simulink model "TST_CoETS_TrqCalc"  (R2016b)
settings: Solver=FixedStepDiscrete  StartTime=0.0  StopTime=simTime  FixedStep=sampleTime  RelTol=1e-3
values from neighbouring files (symbols this model uses):
  testCase = 1    [initTST_CoETS_TrqCalc_001.m]    (also in initTST_CoETS_TrqCalc_002.m = 2; initTST_CoETS_TrqCalc_003.m = 3)
libraries: simulink x52, UnitTest_Lib x48
(part 1 of 2)
settings Model: Creator=zhengjinyan  LastModifiedBy=zhengjinyan
settings DebuggingCC: SignalRangeChecking=error

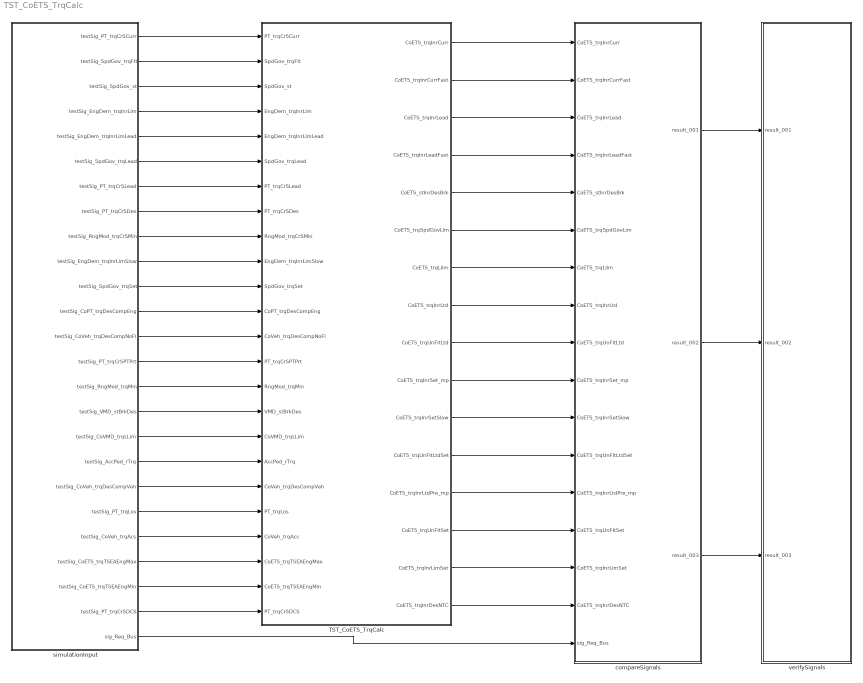
== system TST_CoETS_TrqCalc ==
  TST_CoETS_TrqCalc : Subsystem
  compareSignals : Subsystem
  simulationInput : Subsystem
  verifySignals : Subsystem
  wires:
  simulationInput/1(testSig_PT_trqCrSCurr) -> TST_CoETS_TrqCalc/1(PT_trqCrSCurr)
  simulationInput/2(testSig_SpdGov_trqFlt) -> TST_CoETS_TrqCalc/2(SpdGov_trqFlt)
  simulationInput/3(testSig_SpdGov_st) -> TST_CoETS_TrqCalc/3(SpdGov_st)
  simulationInput/4(testSig_EngDem_trqInrLim) -> TST_CoETS_TrqCalc/4(EngDem_trqInrLim)
  simulationInput/5(testSig_EngDem_trqInrLimLead) -> TST_CoETS_TrqCalc/5(EngDem_trqInrLimLead)
  simulationInput/6(testSig_SpdGov_trqLead) -> TST_CoETS_TrqCalc/6(SpdGov_trqLead)
  simulationInput/7(testSig_PT_trqCrSLead) -> TST_CoETS_TrqCalc/7(PT_trqCrSLead)
  simulationInput/8(testSig_PT_trqCrSDes) -> TST_CoETS_TrqCalc/8(PT_trqCrSDes)
  simulationInput/9(testSig_RngMod_trqCrSMin) -> TST_CoETS_TrqCalc/9(RngMod_trqCrSMin)
  simulationInput/10(testSig_EngDem_trqInrLimSlow) -> TST_CoETS_TrqCalc/10(EngDem_trqInrLimSlow)
  simulationInput/11(testSig_SpdGov_trqSet) -> TST_CoETS_TrqCalc/11(SpdGov_trqSet)
  simulationInput/12(testSig_CoPT_trqDesCompEng) -> TST_CoETS_TrqCalc/12(CoPT_trqDesCompEng)
  simulationInput/13(testSig_CoVeh_trqDesCompNoFl) -> TST_CoETS_TrqCalc/13(CoVeh_trqDesCompNoFl)
  simulationInput/14(testSig_PT_trqCrSPTPrt) -> TST_CoETS_TrqCalc/14(PT_trqCrSPTPrt)
  simulationInput/15(testSig_RngMod_trqMin) -> TST_CoETS_TrqCalc/15(RngMod_trqMin)
  simulationInput/16(testSig_VMD_stBrkDes) -> TST_CoETS_TrqCalc/16(VMD_stBrkDes)
  simulationInput/17(testSig_CoVMD_trqLLim) -> TST_CoETS_TrqCalc/17(CoVMD_trqLLim)
  simulationInput/18(testSig_AccPed_rTrq) -> TST_CoETS_TrqCalc/18(AccPed_rTrq)
  simulationInput/19(testSig_CoVeh_trqDesCompVeh) -> TST_CoETS_TrqCalc/19(CoVeh_trqDesCompVeh)
  simulationInput/20(testSig_PT_trqLos) -> TST_CoETS_TrqCalc/20(PT_trqLos)
  simulationInput/21(testSig_CoVeh_trqAcs) -> TST_CoETS_TrqCalc/21(CoVeh_trqAcs)
  simulationInput/22(testSig_CoETS_trqTSEAEngMax) -> TST_CoETS_TrqCalc/22(CoETS_trqTSEAEngMax)
  simulationInput/23(testSig_CoETS_trqTSEAEngMin) -> TST_CoETS_TrqCalc/23(CoETS_trqTSEAEngMin)
  simulationInput/24(testSig_PT_trqCrSDCS) -> TST_CoETS_TrqCalc/24(PT_trqCrSDCS)
  TST_CoETS_TrqCalc/1(CoETS_trqInrCurr) -> compareSignals/1(CoETS_trqInrCurr)
  TST_CoETS_TrqCalc/2(CoETS_trqInrCurrFast) -> compareSignals/2(CoETS_trqInrCurrFast)
  TST_CoETS_TrqCalc/3(CoETS_trqInrLead) -> compareSignals/3(CoETS_trqInrLead)
  TST_CoETS_TrqCalc/4(CoETS_trqInrLeadFast) -> compareSignals/4(CoETS_trqInrLeadFast)
  TST_CoETS_TrqCalc/5(CoETS_stInrDesBrk) -> compareSignals/5(CoETS_stInrDesBrk)
  TST_CoETS_TrqCalc/6(CoETS_trqSpdGovLim) -> compareSignals/6(CoETS_trqSpdGovLim)
  TST_CoETS_TrqCalc/7(CoETS_trqLlim) -> compareSignals/7(CoETS_trqLlim)
  TST_CoETS_TrqCalc/8(CoETS_trqInrLtd) -> compareSignals/8(CoETS_trqInrLtd)
  TST_CoETS_TrqCalc/9(CoETS_trqUnFltLtd) -> compareSignals/9(CoETS_trqUnFltLtd)
  TST_CoETS_TrqCalc/10(CoETS_trqInrSet_mp) -> compareSignals/10(CoETS_trqInrSet_mp)
  TST_CoETS_TrqCalc/11(CoETS_trqInrSetSlow) -> compareSignals/11(CoETS_trqInrSetSlow)
  TST_CoETS_TrqCalc/12(CoETS_trqUnFltLtdSet) -> compareSignals/12(CoETS_trqUnFltLtdSet)
  TST_CoETS_TrqCalc/13(CoETS_trqInrLtdPre_mp) -> compareSignals/13(CoETS_trqInrLtdPre_mp)
  TST_CoETS_TrqCalc/14(CoETS_trqUnFltSet) -> compareSignals/14(CoETS_trqUnFltSet)
  TST_CoETS_TrqCalc/15(CoETS_trqInrLimSet) -> compareSignals/15(CoETS_trqInrLimSet)
  TST_CoETS_TrqCalc/16(CoETS_trqInrDesNTC) -> compareSignals/16(CoETS_trqInrDesNTC)
  simulationInput/25(sig_Req_Bus) -> compareSignals/17(sig_Req_Bus)
  compareSignals/1(result_001) -> verifySignals/1(result_001)
  compareSignals/2(result_002) -> verifySignals/2(result_002)
  compareSignals/3(result_003) -> verifySignals/3(result_003)

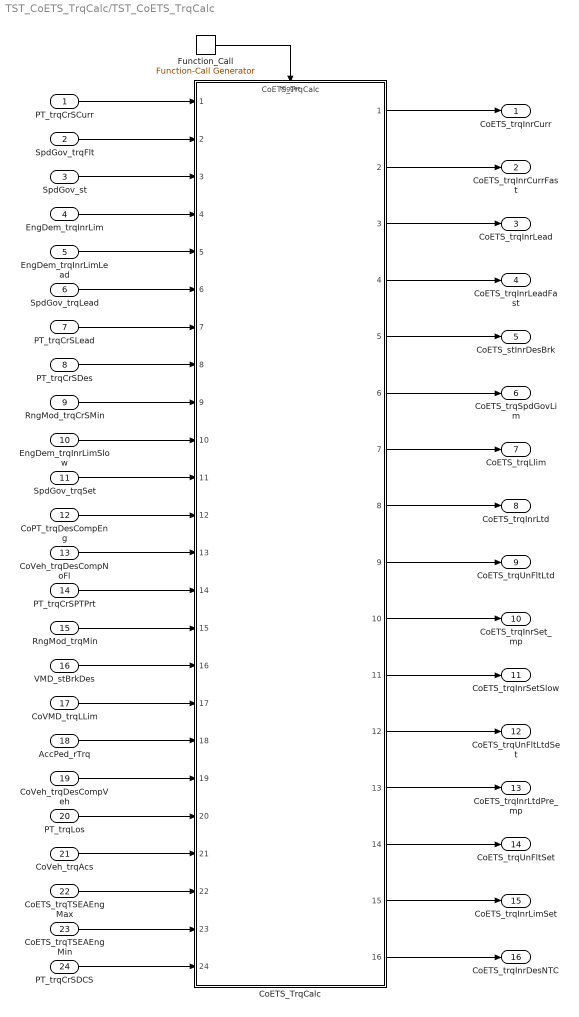
== system TST_CoETS_TrqCalc/TST_CoETS_TrqCalc ==
  PT_trqCrSCurr : Inport
  SpdGov_trqFlt : Inport  Port=2
  SpdGov_st : Inport  Port=3
  EngDem_trqInrLim : Inport  Port=4
  EngDem_trqInrLimLead : Inport  Port=5
  SpdGov_trqLead : Inport  Port=6
  PT_trqCrSLead : Inport  Port=7
  PT_trqCrSDes : Inport  Port=8
  RngMod_trqCrSMin : Inport  Port=9
  EngDem_trqInrLimSlow : Inport  Port=10
  SpdGov_trqSet : Inport  Port=11
  CoPT_trqDesCompEng : Inport  Port=12
  CoVeh_trqDesCompNoFl : Inport  Port=13
  PT_trqCrSPTPrt : Inport  Port=14
  RngMod_trqMin : Inport  Port=15
  VMD_stBrkDes : Inport  Port=16
  CoVMD_trqLLim : Inport  Port=17
  AccPed_rTrq : Inport  Port=18
  CoVeh_trqDesCompVeh : Inport  Port=19
  PT_trqLos : Inport  Port=20
  CoVeh_trqAcs : Inport  Port=21
  CoETS_trqTSEAEngMax : Inport  Port=22
  CoETS_trqTSEAEngMin : Inport  Port=23
  PT_trqCrSDCS : Inport  Port=24
  CoETS_TrqCalc : ModelReference  ModelNameDialog=CoETS_TrqCalc  SimulationMode=Normal  ModelReferenceVersion=1.10  TriggerPortName=function  TriggerPortTriggerType=function-call  TriggerPortStatesWhenEnabling=held
  Function_Call : simulink/Ports & Subsystems/Function-Call Generator  sample_time=sampleTime  numberOfIterations=1
  CoETS_trqInrCurr : Outport
  CoETS_trqInrCurrFast : Outport  Port=2
  CoETS_trqInrLead : Outport  Port=3
  CoETS_trqInrLeadFast : Outport  Port=4
  CoETS_stInrDesBrk : Outport  Port=5
  CoETS_trqSpdGovLim : Outport  Port=6
  CoETS_trqLlim : Outport  Port=7
  CoETS_trqInrLtd : Outport  Port=8
  CoETS_trqUnFltLtd : Outport  Port=9
  CoETS_trqInrSet_mp : Outport  Port=10
  CoETS_trqInrSetSlow : Outport  Port=11
  CoETS_trqUnFltLtdSet : Outport  Port=12
  CoETS_trqInrLtdPre_mp : Outport  Port=13
  CoETS_trqUnFltSet : Outport  Port=14
  CoETS_trqInrLimSet : Outport  Port=15
  CoETS_trqInrDesNTC : Outport  Port=16
  wires:
  Function_Call/1 -> CoETS_TrqCalc/Trigger
  PT_trqCrSCurr/1 -> CoETS_TrqCalc/1
  SpdGov_trqFlt/1 -> CoETS_TrqCalc/2
  SpdGov_st/1 -> CoETS_TrqCalc/3
  EngDem_trqInrLim/1 -> CoETS_TrqCalc/4
  EngDem_trqInrLimLead/1 -> CoETS_TrqCalc/5
  SpdGov_trqLead/1 -> CoETS_TrqCalc/6
  PT_trqCrSLead/1 -> CoETS_TrqCalc/7
  PT_trqCrSDes/1 -> CoETS_TrqCalc/8
  RngMod_trqCrSMin/1 -> CoETS_TrqCalc/9
  EngDem_trqInrLimSlow/1 -> CoETS_TrqCalc/10
  SpdGov_trqSet/1 -> CoETS_TrqCalc/11
  CoPT_trqDesCompEng/1 -> CoETS_TrqCalc/12
  CoVeh_trqDesCompNoFl/1 -> CoETS_TrqCalc/13
  PT_trqCrSPTPrt/1 -> CoETS_TrqCalc/14
  RngMod_trqMin/1 -> CoETS_TrqCalc/15
  VMD_stBrkDes/1 -> CoETS_TrqCalc/16
  CoVMD_trqLLim/1 -> CoETS_TrqCalc/17
  AccPed_rTrq/1 -> CoETS_TrqCalc/18
  CoVeh_trqDesCompVeh/1 -> CoETS_TrqCalc/19
  PT_trqLos/1 -> CoETS_TrqCalc/20
  CoVeh_trqAcs/1 -> CoETS_TrqCalc/21
  CoETS_trqTSEAEngMax/1 -> CoETS_TrqCalc/22
  CoETS_trqTSEAEngMin/1 -> CoETS_TrqCalc/23
  PT_trqCrSDCS/1 -> CoETS_TrqCalc/24
  CoETS_TrqCalc/1 -> CoETS_trqInrCurr/1
  CoETS_TrqCalc/2 -> CoETS_trqInrCurrFast/1
  CoETS_TrqCalc/3 -> CoETS_trqInrLead/1
  CoETS_TrqCalc/5 -> CoETS_stInrDesBrk/1
  CoETS_TrqCalc/6 -> CoETS_trqSpdGovLim/1
  CoETS_TrqCalc/7 -> CoETS_trqLlim/1
  CoETS_TrqCalc/8 -> CoETS_trqInrLtd/1
  CoETS_TrqCalc/9 -> CoETS_trqUnFltLtd/1
  CoETS_TrqCalc/10 -> CoETS_trqInrSet_mp/1
  CoETS_TrqCalc/11 -> CoETS_trqInrSetSlow/1
  CoETS_TrqCalc/12 -> CoETS_trqUnFltLtdSet/1
  CoETS_TrqCalc/13 -> CoETS_trqInrLtdPre_mp/1
  CoETS_TrqCalc/15 -> CoETS_trqInrLimSet/1
  CoETS_TrqCalc/16 -> CoETS_trqInrDesNTC/1
  CoETS_TrqCalc/4 -> CoETS_trqInrLeadFast/1
  CoETS_TrqCalc/14 -> CoETS_trqUnFltSet/1

== system TST_CoETS_TrqCalc/compareSignals ==
  CoETS_trqInrCurr : Inport
  CoETS_trqInrCurrFast : Inport  Port=2
  CoETS_trqInrLead : Inport  Port=3
  CoETS_trqInrLeadFast : Inport  Port=4
  CoETS_stInrDesBrk : Inport  Port=5
  CoETS_trqSpdGovLim : Inport  Port=6
  CoETS_trqLlim : Inport  Port=7
  CoETS_trqInrLtd : Inport  Port=8
  CoETS_trqUnFltLtd : Inport  Port=9
  CoETS_trqInrSet_mp : Inport  Port=10
  CoETS_trqInrSetSlow : Inport  Port=11
  CoETS_trqUnFltLtdSet : Inport  Port=12
  CoETS_trqInrLtdPre_mp : Inport  Port=13
  CoETS_trqUnFltSet : Inport  Port=14
  CoETS_trqInrLimSet : Inport  Port=15
  CoETS_trqInrDesNTC : Inport  Port=16
  sig_Req_Bus : Inport  Port=17
  BC : BusCreator  Inputs=16
  CTC_001 : simulink/Logic and Bit Operations/Compare To Constant  relop===  const=1  OutDataTypeStr=boolean
  CTC_002 : simulink/Logic and Bit Operations/Compare To Constant  relop===  const=2  OutDataTypeStr=boolean
  CTC_003 : simulink/Logic and Bit Operations/Compare To Constant  relop===  const=3  OutDataTypeStr=boolean
  Requirement_001 : Subsystem
  Requirement_002 : Subsystem
  Requirement_003 : Subsystem
  TC_001 : Constant  Value=testCase
  TC_002 : Constant  Value=testCase
  TC_003 : Constant  Value=testCase
  result_001 : Outport
  result_002 : Outport  Port=2
  result_003 : Outport  Port=3
  wires:
  CoETS_trqInrCurr/1 -> BC/1  "CoETS_trqInrCurr"
  CoETS_trqInrCurrFast/1 -> BC/2  "CoETS_trqInrCurrFast"
  CoETS_trqInrLead/1 -> BC/3  "CoETS_trqInrLead"
  CoETS_trqInrLeadFast/1 -> BC/4  "CoETS_trqInrLeadFast"
  CoETS_stInrDesBrk/1 -> BC/5  "CoETS_stInrDesBrk"
  CoETS_trqSpdGovLim/1 -> BC/6  "CoETS_trqSpdGovLim"
  CoETS_trqLlim/1 -> BC/7  "CoETS_trqLlim"
  CoETS_trqInrLtd/1 -> BC/8  "CoETS_trqInrLtd"
  CoETS_trqUnFltLtd/1 -> BC/9  "CoETS_trqUnFltLtd"
  CoETS_trqInrSet_mp/1 -> BC/10  "CoETS_trqInrSet_mp"
  CoETS_trqInrSetSlow/1 -> BC/11  "CoETS_trqInrSetSlow"
  CoETS_trqUnFltLtdSet/1 -> BC/12  "CoETS_trqUnFltLtdSet"
  CoETS_trqInrLtdPre_mp/1 -> BC/13  "CoETS_trqInrLtdPre_mp"
  CoETS_trqUnFltSet/1 -> BC/14  "CoETS_trqUnFltSet"
  CoETS_trqInrLimSet/1 -> BC/15  "CoETS_trqInrLimSet"
  CoETS_trqInrDesNTC/1 -> BC/16  "CoETS_trqInrDesNTC"
  TC_001/1 -> CTC_001/1
  CTC_001/1 -> Requirement_001/Enable
  sig_Req_Bus/1 -> Requirement_001/2(sig_Req_Bus), Requirement_002/2(sig_Req_Bus), Requirement_003/2(sig_Req_Bus)
  BC/1 -> Requirement_002/1(sig_Result_Bus), Requirement_003/1(sig_Result_Bus), Requirement_001/1(sig_Result_Bus)
  Requirement_001/1(result) -> result_001/1
  TC_002/1 -> CTC_002/1
  CTC_002/1 -> Requirement_002/Enable
  Requirement_002/1(result) -> result_002/1
  TC_003/1 -> CTC_003/1
  CTC_003/1 -> Requirement_003/Enable
  Requirement_003/1(result) -> result_003/1

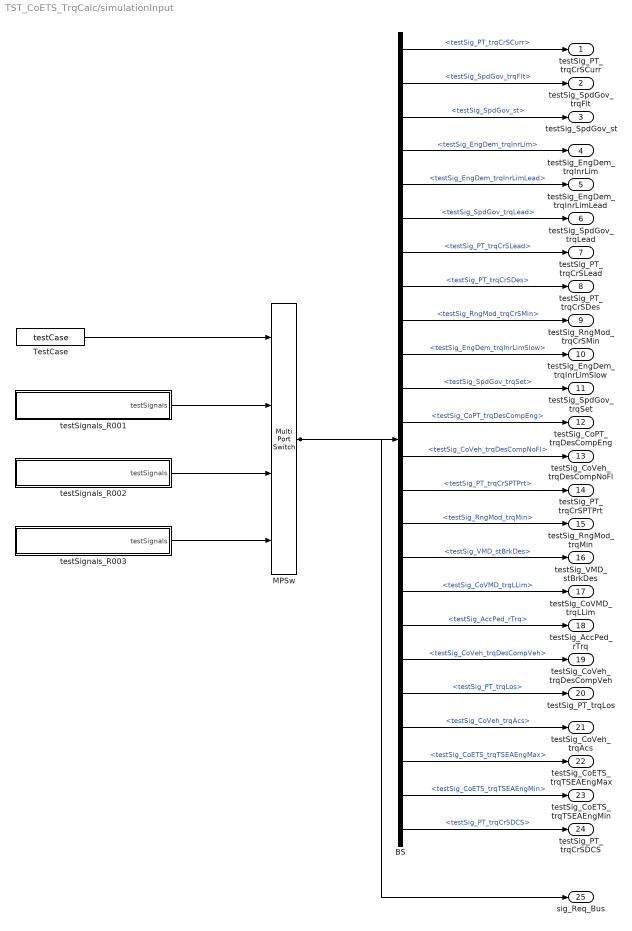
== system TST_CoETS_TrqCalc/simulationInput ==
  BS : BusSelector  OutputSignals=testSig_PT_trqCrSCurr,testSig_SpdGov_trqFlt,testSig_SpdGov_st,testSig_EngDem_trqInrLim,testSig_EngDem_trqInrLimLead,testSig_SpdGov_trqLead,testSig_PT_trqCrSLead,testSig_PT_trqCrSDes,testSig_RngMod_trqCrSMin,testSig_EngDem_trqInrLimSlow,testSig_SpdGov_trqSet,testSig_CoPT_trqDesCompEng,testSig_CoVeh_trqDesCompNoFl,testSig_PT_trqCrSPTPrt,testSig_RngMod_trqMin,testSig_VMD_stBrkDes,testSig_CoVMD_trqLLim,testSig_AccPed_rTrq,testSig_CoVeh_trqDesCompVeh,testSig_PT_trqLos,testSig_CoVeh_trqAcs,testSig_CoETS_trqTSEAEngMax,testSig_CoETS_trqTSEAEngMin,testSig_PT_trqCrSDCS
  MPSw : MultiPortSwitch  SaturateOnIntegerOverflow=on  InputSameDT=on
  TestCase : Constant  Value=testCase
  testSignals_R001 : Subsystem
  testSignals_R002 : Subsystem
  testSignals_R003 : Subsystem
  testSig_PT_trqCrSCurr : Outport
  testSig_SpdGov_trqFlt : Outport  Port=2
  testSig_SpdGov_st : Outport  Port=3
  testSig_EngDem_trqInrLim : Outport  Port=4
  testSig_EngDem_trqInrLimLead : Outport  Port=5
  testSig_SpdGov_trqLead : Outport  Port=6
  testSig_PT_trqCrSLead : Outport  Port=7
  testSig_PT_trqCrSDes : Outport  Port=8
  testSig_RngMod_trqCrSMin : Outport  Port=9
  testSig_EngDem_trqInrLimSlow : Outport  Port=10
  testSig_SpdGov_trqSet : Outport  Port=11
  testSig_CoPT_trqDesCompEng : Outport  Port=12
  testSig_CoVeh_trqDesCompNoFl : Outport  Port=13
  testSig_PT_trqCrSPTPrt : Outport  Port=14
  testSig_RngMod_trqMin : Outport  Port=15
  testSig_VMD_stBrkDes : Outport  Port=16
  testSig_CoVMD_trqLLim : Outport  Port=17
  testSig_AccPed_rTrq : Outport  Port=18
  testSig_CoVeh_trqDesCompVeh : Outport  Port=19
  testSig_PT_trqLos : Outport  Port=20
  testSig_CoVeh_trqAcs : Outport  Port=21
  testSig_CoETS_trqTSEAEngMax : Outport  Port=22
  testSig_CoETS_trqTSEAEngMin : Outport  Port=23
  testSig_PT_trqCrSDCS : Outport  Port=24
  sig_Req_Bus : Outport  Port=25
  wires:
  BS/1 -> testSig_PT_trqCrSCurr/1  "<testSig_PT_trqCrSCurr>"
  BS/2 -> testSig_SpdGov_trqFlt/1  "<testSig_SpdGov_trqFlt>"
  BS/3 -> testSig_SpdGov_st/1  "<testSig_SpdGov_st>"
  BS/4 -> testSig_EngDem_trqInrLim/1  "<testSig_EngDem_trqInrLim>"
  BS/5 -> testSig_EngDem_trqInrLimLead/1  "<testSig_EngDem_trqInrLimLead>"
  BS/6 -> testSig_SpdGov_trqLead/1  "<testSig_SpdGov_trqLead>"
  BS/7 -> testSig_PT_trqCrSLead/1  "<testSig_PT_trqCrSLead>"
  BS/8 -> testSig_PT_trqCrSDes/1  "<testSig_PT_trqCrSDes>"
  BS/9 -> testSig_RngMod_trqCrSMin/1  "<testSig_RngMod_trqCrSMin>"
  BS/10 -> testSig_EngDem_trqInrLimSlow/1  "<testSig_EngDem_trqInrLimSlow>"
  BS/11 -> testSig_SpdGov_trqSet/1  "<testSig_SpdGov_trqSet>"
  BS/12 -> testSig_CoPT_trqDesCompEng/1  "<testSig_CoPT_trqDesCompEng>"
  BS/13 -> testSig_CoVeh_trqDesCompNoFl/1  "<testSig_CoVeh_trqDesCompNoFl>"
  BS/14 -> testSig_PT_trqCrSPTPrt/1  "<testSig_PT_trqCrSPTPrt>"
  BS/15 -> testSig_RngMod_trqMin/1  "<testSig_RngMod_trqMin>"
  BS/16 -> testSig_VMD_stBrkDes/1  "<testSig_VMD_stBrkDes>"
  BS/17 -> testSig_CoVMD_trqLLim/1  "<testSig_CoVMD_trqLLim>"
  BS/18 -> testSig_AccPed_rTrq/1  "<testSig_AccPed_rTrq>"
  BS/19 -> testSig_CoVeh_trqDesCompVeh/1  "<testSig_CoVeh_trqDesCompVeh>"
  BS/20 -> testSig_PT_trqLos/1  "<testSig_PT_trqLos>"
  BS/21 -> testSig_CoVeh_trqAcs/1  "<testSig_CoVeh_trqAcs>"
  BS/22 -> testSig_CoETS_trqTSEAEngMax/1  "<testSig_CoETS_trqTSEAEngMax>"
  BS/23 -> testSig_CoETS_trqTSEAEngMin/1  "<testSig_CoETS_trqTSEAEngMin>"
  BS/24 -> testSig_PT_trqCrSDCS/1  "<testSig_PT_trqCrSDCS>"
  MPSw/1 -> BS/1, sig_Req_Bus/1
  TestCase/1 -> MPSw/1
  testSignals_R001/1(testSignals) -> MPSw/2
  testSignals_R002/1(testSignals) -> MPSw/3
  testSignals_R003/1(testSignals) -> MPSw/4

== system TST_CoETS_TrqCalc/verifySignals ==
  result_001 : Inport
  result_002 : Inport  Port=2
  result_003 : Inport  Port=3
  Assertion_001 : Assertion  Enabled=off
  Assertion_002 : Assertion  Enabled=off
  Assertion_003 : Assertion  Enabled=off
  wires:
  result_001/1 -> Assertion_001/1
  result_002/1 -> Assertion_002/1
  result_003/1 -> Assertion_003/1

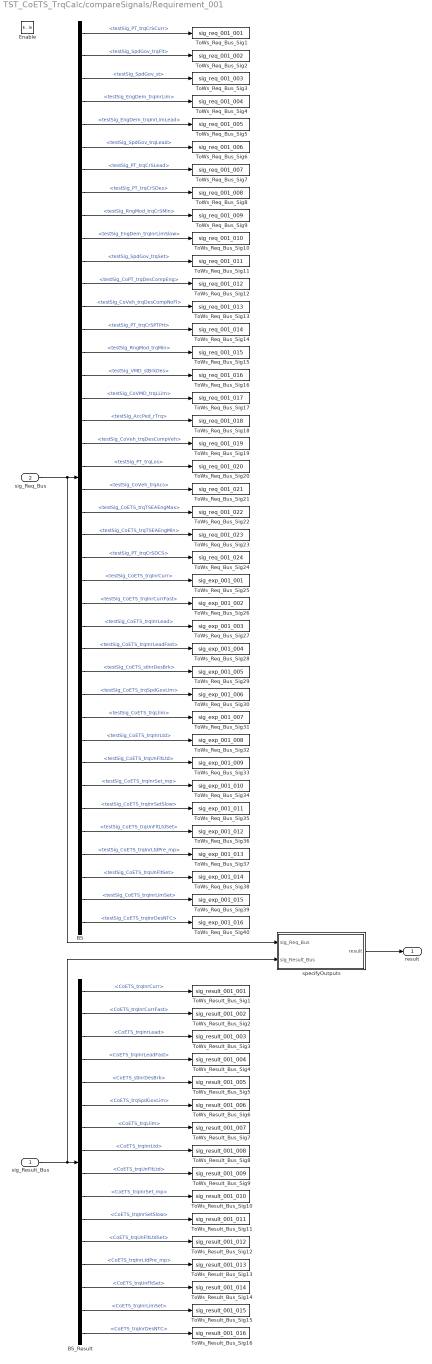
== system TST_CoETS_TrqCalc/compareSignals/Requirement_001 ==
  sig_Result_Bus : Inport
  sig_Req_Bus : Inport  Port=2
  Enable : EnablePort
  BS : BusSelector  OutputSignals=testSig_PT_trqCrSCurr,testSig_SpdGov_trqFlt,testSig_SpdGov_st,testSig_EngDem_trqInrLim,testSig_EngDem_trqInrLimLead,testSig_SpdGov_trqLead,testSig_PT_trqCrSLead,testSig_PT_trqCrSDes,testSig_RngMod_trqCrSMin,testSig_EngDem_trqInrLimSlow,testSig_SpdGov_trqSet,testSig_CoPT_trqDesCompEng,testSig_CoVeh_trqDesCompNoFl,testSig_PT_trqCrSPTPrt,testSig_RngMod_trqMin,testSig_VMD_stBrkDes,testSig_CoVMD_trqLLim,testSig_AccPed_rTrq,testSig_CoVeh_trqDesCompVeh,testSig_PT_trqLos,testSig_CoVeh_trqAcs,testSig_CoETS_trqTSEAEngMax,testSig_CoETS_trqTSEAEngMin,testSig_PT_trqCrSDCS,testSig_CoETS_trqInrCurr,testSig_CoETS_trqInrCurrFast,testSig_CoETS_trqInrLead,testSig_CoETS_trqInrLeadFast,testSig_CoETS_stInrDesBrk,testSig_CoETS_trqSpdGovLim,testSig_CoETS_trqLlim,testSig_CoETS_trqInrLtd,testSig_CoETS_trqUnFltLtd,testSig_CoETS_trqInrSet_mp,testSig_CoETS_trqInrSetSlow,testSig_CoETS_trqUnFltLtdSet,testSig_CoETS_trqInrLtdPre_mp,testSig_CoETS_trqUnFltSet,testSig_CoETS_trqInrLimSet,testSig_CoETS_trqInrDesNTC
  BS_Result : BusSelector  OutputSignals=CoETS_trqInrCurr,CoETS_trqInrCurrFast,CoETS_trqInrLead,CoETS_trqInrLeadFast,CoETS_stInrDesBrk,CoETS_trqSpdGovLim,CoETS_trqLlim,CoETS_trqInrLtd,CoETS_trqUnFltLtd,CoETS_trqInrSet_mp,CoETS_trqInrSetSlow,CoETS_trqUnFltLtdSet,CoETS_trqInrLtdPre_mp,CoETS_trqUnFltSet,CoETS_trqInrLimSet,CoETS_trqInrDesNTC
  ToWs_Req_Bus_Sig1 : ToWorkspace  VariableName=sig_req_001_001  SaveFormat=Structure With Time
  ToWs_Req_Bus_Sig10 : ToWorkspace  VariableName=sig_req_001_010  SaveFormat=Structure With Time
  ToWs_Req_Bus_Sig11 : ToWorkspace  VariableName=sig_req_001_011  SaveFormat=Structure With Time
  ToWs_Req_Bus_Sig12 : ToWorkspace  VariableName=sig_req_001_012  SaveFormat=Structure With Time
  ToWs_Req_Bus_Sig13 : ToWorkspace  VariableName=sig_req_001_013  SaveFormat=Structure With Time
  ToWs_Req_Bus_Sig14 : ToWorkspace  VariableName=sig_req_001_014  SaveFormat=Structure With Time
  ToWs_Req_Bus_Sig15 : ToWorkspace  VariableName=sig_req_001_015  SaveFormat=Structure With Time
  ToWs_Req_Bus_Sig16 : ToWorkspace  VariableName=sig_req_001_016  SaveFormat=Structure With Time
  ToWs_Req_Bus_Sig17 : ToWorkspace  VariableName=sig_req_001_017  SaveFormat=Structure With Time
  ToWs_Req_Bus_Sig18 : ToWorkspace  VariableName=sig_req_001_018  SaveFormat=Structure With Time
  ToWs_Req_Bus_Sig19 : ToWorkspace  VariableName=sig_req_001_019  SaveFormat=Structure With Time
  ToWs_Req_Bus_Sig2 : ToWorkspace  VariableName=sig_req_001_002  SaveFormat=Structure With Time
  ToWs_Req_Bus_Sig20 : ToWorkspace  VariableName=sig_req_001_020  SaveFormat=Structure With Time
  ToWs_Req_Bus_Sig21 : ToWorkspace  VariableName=sig_req_001_021  SaveFormat=Structure With Time
  ToWs_Req_Bus_Sig22 : ToWorkspace  VariableName=sig_req_001_022  SaveFormat=Structure With Time
  ToWs_Req_Bus_Sig23 : ToWorkspace  VariableName=sig_req_001_023  SaveFormat=Structure With Time
  ToWs_Req_Bus_Sig24 : ToWorkspace  VariableName=sig_req_001_024  SaveFormat=Structure With Time
  ToWs_Req_Bus_Sig25 : ToWorkspace  VariableName=sig_exp_001_001  SaveFormat=Structure With Time
  ToWs_Req_Bus_Sig26 : ToWorkspace  VariableName=sig_exp_001_002  SaveFormat=Structure With Time
  ToWs_Req_Bus_Sig27 : ToWorkspace  VariableName=sig_exp_001_003  SaveFormat=Structure With Time
  ToWs_Req_Bus_Sig28 : ToWorkspace  VariableName=sig_exp_001_004  SaveFormat=Structure With Time
  ToWs_Req_Bus_Sig29 : ToWorkspace  VariableName=sig_exp_001_005  SaveFormat=Structure With Time
  ToWs_Req_Bus_Sig3 : ToWorkspace  VariableName=sig_req_001_003  SaveFormat=Structure With Time
  ToWs_Req_Bus_Sig30 : ToWorkspace  VariableName=sig_exp_001_006  SaveFormat=Structure With Time
  ToWs_Req_Bus_Sig31 : ToWorkspace  VariableName=sig_exp_001_007  SaveFormat=Structure With Time
  ToWs_Req_Bus_Sig32 : ToWorkspace  VariableName=sig_exp_001_008  SaveFormat=Structure With Time
  ToWs_Req_Bus_Sig33 : ToWorkspace  VariableName=sig_exp_001_009  SaveFormat=Structure With Time
  ToWs_Req_Bus_Sig34 : ToWorkspace  VariableName=sig_exp_001_010  SaveFormat=Structure With Time
  ToWs_Req_Bus_Sig35 : ToWorkspace  VariableName=sig_exp_001_011  SaveFormat=Structure With Time
  ToWs_Req_Bus_Sig36 : ToWorkspace  VariableName=sig_exp_001_012  SaveFormat=Structure With Time
  ToWs_Req_Bus_Sig37 : ToWorkspace  VariableName=sig_exp_001_013  SaveFormat=Structure With Time
  ToWs_Req_Bus_Sig38 : ToWorkspace  VariableName=sig_exp_001_014  SaveFormat=Structure With Time
  ToWs_Req_Bus_Sig39 : ToWorkspace  VariableName=sig_exp_001_015  SaveFormat=Structure With Time
  ToWs_Req_Bus_Sig4 : ToWorkspace  VariableName=sig_req_001_004  SaveFormat=Structure With Time
  ToWs_Req_Bus_Sig40 : ToWorkspace  VariableName=sig_exp_001_016  SaveFormat=Structure With Time
  ToWs_Req_Bus_Sig5 : ToWorkspace  VariableName=sig_req_001_005  SaveFormat=Structure With Time
  ToWs_Req_Bus_Sig6 : ToWorkspace  VariableName=sig_req_001_006  SaveFormat=Structure With Time
  ToWs_Req_Bus_Sig7 : ToWorkspace  VariableName=sig_req_001_007  SaveFormat=Structure With Time
  ToWs_Req_Bus_Sig8 : ToWorkspace  VariableName=sig_req_001_008  SaveFormat=Structure With Time
  ToWs_Req_Bus_Sig9 : ToWorkspace  VariableName=sig_req_001_009  SaveFormat=Structure With Time
  ToWs_Result_Bus_Sig1 : ToWorkspace  VariableName=sig_result_001_001  SaveFormat=Structure With Time
  ToWs_Result_Bus_Sig10 : ToWorkspace  VariableName=sig_result_001_010  SaveFormat=Structure With Time
  ToWs_Result_Bus_Sig11 : ToWorkspace  VariableName=sig_result_001_011  SaveFormat=Structure With Time
  ToWs_Result_Bus_Sig12 : ToWorkspace  VariableName=sig_result_001_012  SaveFormat=Structure With Time
  ToWs_Result_Bus_Sig13 : ToWorkspace  VariableName=sig_result_001_013  SaveFormat=Structure With Time
  ToWs_Result_Bus_Sig14 : ToWorkspace  VariableName=sig_result_001_014  SaveFormat=Structure With Time
  ToWs_Result_Bus_Sig15 : ToWorkspace  VariableName=sig_result_001_015  SaveFormat=Structure With Time
  ToWs_Result_Bus_Sig16 : ToWorkspace  VariableName=sig_result_001_016  SaveFormat=Structure With Time
  ToWs_Result_Bus_Sig2 : ToWorkspace  VariableName=sig_result_001_002  SaveFormat=Structure With Time
  ToWs_Result_Bus_Sig3 : ToWorkspace  VariableName=sig_result_001_003  SaveFormat=Structure With Time
  ToWs_Result_Bus_Sig4 : ToWorkspace  VariableName=sig_result_001_004  SaveFormat=Structure With Time
  ToWs_Result_Bus_Sig5 : ToWorkspace  VariableName=sig_result_001_005  SaveFormat=Structure With Time
  ToWs_Result_Bus_Sig6 : ToWorkspace  VariableName=sig_result_001_006  SaveFormat=Structure With Time
  ToWs_Result_Bus_Sig7 : ToWorkspace  VariableName=sig_result_001_007  SaveFormat=Structure With Time
  ToWs_Result_Bus_Sig8 : ToWorkspace  VariableName=sig_result_001_008  SaveFormat=Structure With Time
  ToWs_Result_Bus_Sig9 : ToWorkspace  VariableName=sig_result_001_009  SaveFormat=Structure With Time
  specifyOutputs : Subsystem
  result : Outport
  wires:
  sig_Req_Bus/1 -> BS/1, specifyOutputs/1(sig_Req_Bus)
  BS/1 -> ToWs_Req_Bus_Sig1/1  "<testSig_PT_trqCrSCurr>"
  BS/2 -> ToWs_Req_Bus_Sig2/1  "<testSig_SpdGov_trqFlt>"
  BS/3 -> ToWs_Req_Bus_Sig3/1  "<testSig_SpdGov_st>"
  BS/4 -> ToWs_Req_Bus_Sig4/1  "<testSig_EngDem_trqInrLim>"
  BS/5 -> ToWs_Req_Bus_Sig5/1  "<testSig_EngDem_trqInrLimLead>"
  BS/6 -> ToWs_Req_Bus_Sig6/1  "<testSig_SpdGov_trqLead>"
  BS/7 -> ToWs_Req_Bus_Sig7/1  "<testSig_PT_trqCrSLead>"
  BS/8 -> ToWs_Req_Bus_Sig8/1  "<testSig_PT_trqCrSDes>"
  BS/9 -> ToWs_Req_Bus_Sig9/1  "<testSig_RngMod_trqCrSMin>"
  BS/10 -> ToWs_Req_Bus_Sig10/1  "<testSig_EngDem_trqInrLimSlow>"
  BS/11 -> ToWs_Req_Bus_Sig11/1  "<testSig_SpdGov_trqSet>"
  BS/12 -> ToWs_Req_Bus_Sig12/1  "<testSig_CoPT_trqDesCompEng>"
  BS/13 -> ToWs_Req_Bus_Sig13/1  "<testSig_CoVeh_trqDesCompNoFl>"
  BS/14 -> ToWs_Req_Bus_Sig14/1  "<testSig_PT_trqCrSPTPrt>"
  BS/15 -> ToWs_Req_Bus_Sig15/1  "<testSig_RngMod_trqMin>"
  BS/16 -> ToWs_Req_Bus_Sig16/1  "<testSig_VMD_stBrkDes>"
  BS/17 -> ToWs_Req_Bus_Sig17/1  "<testSig_CoVMD_trqLLim>"
  BS/18 -> ToWs_Req_Bus_Sig18/1  "<testSig_AccPed_rTrq>"
  BS/19 -> ToWs_Req_Bus_Sig19/1  "<testSig_CoVeh_trqDesCompVeh>"
  BS/20 -> ToWs_Req_Bus_Sig20/1  "<testSig_PT_trqLos>"
  BS/21 -> ToWs_Req_Bus_Sig21/1  "<testSig_CoVeh_trqAcs>"
  BS/22 -> ToWs_Req_Bus_Sig22/1  "<testSig_CoETS_trqTSEAEngMax>"
  BS/23 -> ToWs_Req_Bus_Sig23/1  "<testSig_CoETS_trqTSEAEngMin>"
  BS/24 -> ToWs_Req_Bus_Sig24/1  "<testSig_PT_trqCrSDCS>"
  BS/25 -> ToWs_Req_Bus_Sig25/1  "<testSig_CoETS_trqInrCurr>"
  BS/26 -> ToWs_Req_Bus_Sig26/1  "<testSig_CoETS_trqInrCurrFast>"
  BS/27 -> ToWs_Req_Bus_Sig27/1  "<testSig_CoETS_trqInrLead>"
  BS/28 -> ToWs_Req_Bus_Sig28/1  "<testSig_CoETS_trqInrLeadFast>"
  BS/29 -> ToWs_Req_Bus_Sig29/1  "<testSig_CoETS_stInrDesBrk>"
  BS/30 -> ToWs_Req_Bus_Sig30/1  "<testSig_CoETS_trqSpdGovLim>"
  BS/31 -> ToWs_Req_Bus_Sig31/1  "<testSig_CoETS_trqLlim>"
  BS/32 -> ToWs_Req_Bus_Sig32/1  "<testSig_CoETS_trqInrLtd>"
  BS/33 -> ToWs_Req_Bus_Sig33/1  "<testSig_CoETS_trqUnFltLtd>"
  BS/34 -> ToWs_Req_Bus_Sig34/1  "<testSig_CoETS_trqInrSet_mp>"
  BS/35 -> ToWs_Req_Bus_Sig35/1  "<testSig_CoETS_trqInrSetSlow>"
  BS/36 -> ToWs_Req_Bus_Sig36/1  "<testSig_CoETS_trqUnFltLtdSet>"
  BS/37 -> ToWs_Req_Bus_Sig37/1  "<testSig_CoETS_trqInrLtdPre_mp>"
  BS/38 -> ToWs_Req_Bus_Sig38/1  "<testSig_CoETS_trqUnFltSet>"
  BS/39 -> ToWs_Req_Bus_Sig39/1  "<testSig_CoETS_trqInrLimSet>"
  BS/40 -> ToWs_Req_Bus_Sig40/1  "<testSig_CoETS_trqInrDesNTC>"
  sig_Result_Bus/1 -> BS_Result/1, specifyOutputs/2(sig_Result_Bus)
  BS_Result/1 -> ToWs_Result_Bus_Sig1/1  "<CoETS_trqInrCurr>"
  BS_Result/2 -> ToWs_Result_Bus_Sig2/1  "<CoETS_trqInrCurrFast>"
  BS_Result/3 -> ToWs_Result_Bus_Sig3/1  "<CoETS_trqInrLead>"
  BS_Result/4 -> ToWs_Result_Bus_Sig4/1  "<CoETS_trqInrLeadFast>"
  BS_Result/5 -> ToWs_Result_Bus_Sig5/1  "<CoETS_stInrDesBrk>"
  BS_Result/6 -> ToWs_Result_Bus_Sig6/1  "<CoETS_trqSpdGovLim>"
  BS_Result/7 -> ToWs_Result_Bus_Sig7/1  "<CoETS_trqLlim>"
  BS_Result/8 -> ToWs_Result_Bus_Sig8/1  "<CoETS_trqInrLtd>"
  BS_Result/9 -> ToWs_Result_Bus_Sig9/1  "<CoETS_trqUnFltLtd>"
  BS_Result/10 -> ToWs_Result_Bus_Sig10/1  "<CoETS_trqInrSet_mp>"
  BS_Result/11 -> ToWs_Result_Bus_Sig11/1  "<CoETS_trqInrSetSlow>"
  BS_Result/12 -> ToWs_Result_Bus_Sig12/1  "<CoETS_trqUnFltLtdSet>"
  BS_Result/13 -> ToWs_Result_Bus_Sig13/1  "<CoETS_trqInrLtdPre_mp>"
  BS_Result/14 -> ToWs_Result_Bus_Sig14/1  "<CoETS_trqUnFltSet>"
  BS_Result/15 -> ToWs_Result_Bus_Sig15/1  "<CoETS_trqInrLimSet>"
  BS_Result/16 -> ToWs_Result_Bus_Sig16/1  "<CoETS_trqInrDesNTC>"
  specifyOutputs/1(result) -> result/1

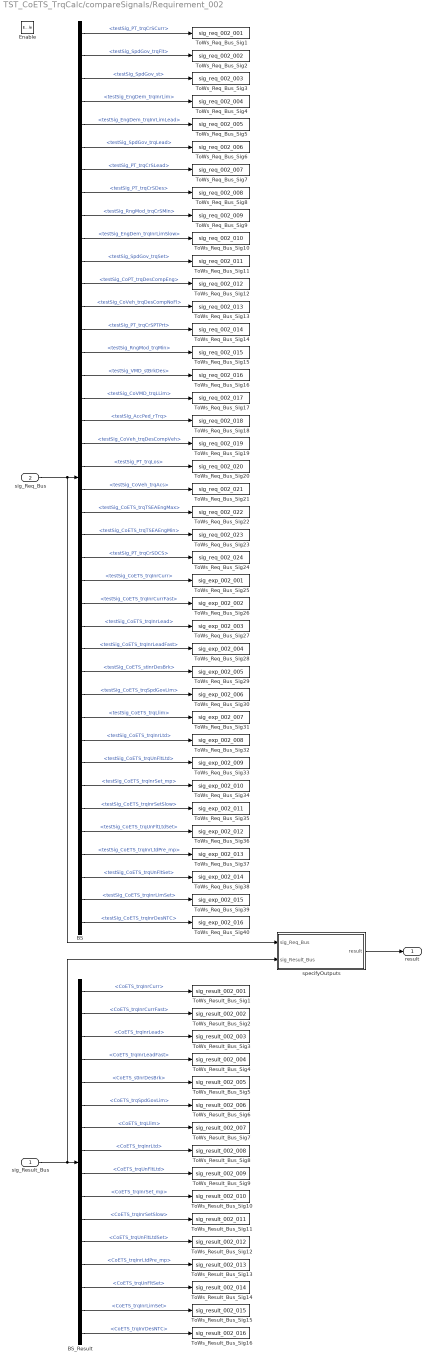
== system TST_CoETS_TrqCalc/compareSignals/Requirement_002 ==
  sig_Result_Bus : Inport
  sig_Req_Bus : Inport  Port=2
  Enable : EnablePort
  BS : BusSelector  OutputSignals=testSig_PT_trqCrSCurr,testSig_SpdGov_trqFlt,testSig_SpdGov_st,testSig_EngDem_trqInrLim,testSig_EngDem_trqInrLimLead,testSig_SpdGov_trqLead,testSig_PT_trqCrSLead,testSig_PT_trqCrSDes,testSig_RngMod_trqCrSMin,testSig_EngDem_trqInrLimSlow,testSig_SpdGov_trqSet,testSig_CoPT_trqDesCompEng,testSig_CoVeh_trqDesCompNoFl,testSig_PT_trqCrSPTPrt,testSig_RngMod_trqMin,testSig_VMD_stBrkDes,testSig_CoVMD_trqLLim,testSig_AccPed_rTrq,testSig_CoVeh_trqDesCompVeh,testSig_PT_trqLos,testSig_CoVeh_trqAcs,testSig_CoETS_trqTSEAEngMax,testSig_CoETS_trqTSEAEngMin,testSig_PT_trqCrSDCS,testSig_CoETS_trqInrCurr,testSig_CoETS_trqInrCurrFast,testSig_CoETS_trqInrLead,testSig_CoETS_trqInrLeadFast,testSig_CoETS_stInrDesBrk,testSig_CoETS_trqSpdGovLim,testSig_CoETS_trqLlim,testSig_CoETS_trqInrLtd,testSig_CoETS_trqUnFltLtd,testSig_CoETS_trqInrSet_mp,testSig_CoETS_trqInrSetSlow,testSig_CoETS_trqUnFltLtdSet,testSig_CoETS_trqInrLtdPre_mp,testSig_CoETS_trqUnFltSet,testSig_CoETS_trqInrLimSet,testSig_CoETS_trqInrDesNTC
  BS_Result : BusSelector  OutputSignals=CoETS_trqInrCurr,CoETS_trqInrCurrFast,CoETS_trqInrLead,CoETS_trqInrLeadFast,CoETS_stInrDesBrk,CoETS_trqSpdGovLim,CoETS_trqLlim,CoETS_trqInrLtd,CoETS_trqUnFltLtd,CoETS_trqInrSet_mp,CoETS_trqInrSetSlow,CoETS_trqUnFltLtdSet,CoETS_trqInrLtdPre_mp,CoETS_trqUnFltSet,CoETS_trqInrLimSet,CoETS_trqInrDesNTC
  ToWs_Req_Bus_Sig1 : ToWorkspace  VariableName=sig_req_002_001  SaveFormat=Structure With Time
  ToWs_Req_Bus_Sig10 : ToWorkspace  VariableName=sig_req_002_010  SaveFormat=Structure With Time
  ToWs_Req_Bus_Sig11 : ToWorkspace  VariableName=sig_req_002_011  SaveFormat=Structure With Time
  ToWs_Req_Bus_Sig12 : ToWorkspace  VariableName=sig_req_002_012  SaveFormat=Structure With Time
  ToWs_Req_Bus_Sig13 : ToWorkspace  VariableName=sig_req_002_013  SaveFormat=Structure With Time
  ToWs_Req_Bus_Sig14 : ToWorkspace  VariableName=sig_req_002_014  SaveFormat=Structure With Time
  ToWs_Req_Bus_Sig15 : ToWorkspace  VariableName=sig_req_002_015  SaveFormat=Structure With Time
  ToWs_Req_Bus_Sig16 : ToWorkspace  VariableName=sig_req_002_016  SaveFormat=Structure With Time
  ToWs_Req_Bus_Sig17 : ToWorkspace  VariableName=sig_req_002_017  SaveFormat=Structure With Time
  ToWs_Req_Bus_Sig18 : ToWorkspace  VariableName=sig_req_002_018  SaveFormat=Structure With Time
  ToWs_Req_Bus_Sig19 : ToWorkspace  VariableName=sig_req_002_019  SaveFormat=Structure With Time
  ToWs_Req_Bus_Sig2 : ToWorkspace  VariableName=sig_req_002_002  SaveFormat=Structure With Time
  ToWs_Req_Bus_Sig20 : ToWorkspace  VariableName=sig_req_002_020  SaveFormat=Structure With Time
  ToWs_Req_Bus_Sig21 : ToWorkspace  VariableName=sig_req_002_021  SaveFormat=Structure With Time
  ToWs_Req_Bus_Sig22 : ToWorkspace  VariableName=sig_req_002_022  SaveFormat=Structure With Time
  ToWs_Req_Bus_Sig23 : ToWorkspace  VariableName=sig_req_002_023  SaveFormat=Structure With Time
  ToWs_Req_Bus_Sig24 : ToWorkspace  VariableName=sig_req_002_024  SaveFormat=Structure With Time
  ToWs_Req_Bus_Sig25 : ToWorkspace  VariableName=sig_exp_002_001  SaveFormat=Structure With Time
  ToWs_Req_Bus_Sig26 : ToWorkspace  VariableName=sig_exp_002_002  SaveFormat=Structure With Time
  ToWs_Req_Bus_Sig27 : ToWorkspace  VariableName=sig_exp_002_003  SaveFormat=Structure With Time
  ToWs_Req_Bus_Sig28 : ToWorkspace  VariableName=sig_exp_002_004  SaveFormat=Structure With Time
  ToWs_Req_Bus_Sig29 : ToWorkspace  VariableName=sig_exp_002_005  SaveFormat=Structure With Time
  ToWs_Req_Bus_Sig3 : ToWorkspace  VariableName=sig_req_002_003  SaveFormat=Structure With Time
  ToWs_Req_Bus_Sig30 : ToWorkspace  VariableName=sig_exp_002_006  SaveFormat=Structure With Time
  ToWs_Req_Bus_Sig31 : ToWorkspace  VariableName=sig_exp_002_007  SaveFormat=Structure With Time
  ToWs_Req_Bus_Sig32 : ToWorkspace  VariableName=sig_exp_002_008  SaveFormat=Structure With Time
  ToWs_Req_Bus_Sig33 : ToWorkspace  VariableName=sig_exp_002_009  SaveFormat=Structure With Time
  ToWs_Req_Bus_Sig34 : ToWorkspace  VariableName=sig_exp_002_010  SaveFormat=Structure With Time
  ToWs_Req_Bus_Sig35 : ToWorkspace  VariableName=sig_exp_002_011  SaveFormat=Structure With Time
  ToWs_Req_Bus_Sig36 : ToWorkspace  VariableName=sig_exp_002_012  SaveFormat=Structure With Time
  ToWs_Req_Bus_Sig37 : ToWorkspace  VariableName=sig_exp_002_013  SaveFormat=Structure With Time
  ToWs_Req_Bus_Sig38 : ToWorkspace  VariableName=sig_exp_002_014  SaveFormat=Structure With Time
  ToWs_Req_Bus_Sig39 : ToWorkspace  VariableName=sig_exp_002_015  SaveFormat=Structure With Time
  ToWs_Req_Bus_Sig4 : ToWorkspace  VariableName=sig_req_002_004  SaveFormat=Structure With Time
  ToWs_Req_Bus_Sig40 : ToWorkspace  VariableName=sig_exp_002_016  SaveFormat=Structure With Time
  ToWs_Req_Bus_Sig5 : ToWorkspace  VariableName=sig_req_002_005  SaveFormat=Structure With Time
  ToWs_Req_Bus_Sig6 : ToWorkspace  VariableName=sig_req_002_006  SaveFormat=Structure With Time
  ToWs_Req_Bus_Sig7 : ToWorkspace  VariableName=sig_req_002_007  SaveFormat=Structure With Time
  ToWs_Req_Bus_Sig8 : ToWorkspace  VariableName=sig_req_002_008  SaveFormat=Structure With Time
  ToWs_Req_Bus_Sig9 : ToWorkspace  VariableName=sig_req_002_009  SaveFormat=Structure With Time
  ToWs_Result_Bus_Sig1 : ToWorkspace  VariableName=sig_result_002_001  SaveFormat=Structure With Time
  ToWs_Result_Bus_Sig10 : ToWorkspace  VariableName=sig_result_002_010  SaveFormat=Structure With Time
  ToWs_Result_Bus_Sig11 : ToWorkspace  VariableName=sig_result_002_011  SaveFormat=Structure With Time
  ToWs_Result_Bus_Sig12 : ToWorkspace  VariableName=sig_result_002_012  SaveFormat=Structure With Time
  ToWs_Result_Bus_Sig13 : ToWorkspace  VariableName=sig_result_002_013  SaveFormat=Structure With Time
  ToWs_Result_Bus_Sig14 : ToWorkspace  VariableName=sig_result_002_014  SaveFormat=Structure With Time
  ToWs_Result_Bus_Sig15 : ToWorkspace  VariableName=sig_result_002_015  SaveFormat=Structure With Time
  ToWs_Result_Bus_Sig16 : ToWorkspace  VariableName=sig_result_002_016  SaveFormat=Structure With Time
  ToWs_Result_Bus_Sig2 : ToWorkspace  VariableName=sig_result_002_002  SaveFormat=Structure With Time
  ToWs_Result_Bus_Sig3 : ToWorkspace  VariableName=sig_result_002_003  SaveFormat=Structure With Time
  ToWs_Result_Bus_Sig4 : ToWorkspace  VariableName=sig_result_002_004  SaveFormat=Structure With Time
  ToWs_Result_Bus_Sig5 : ToWorkspace  VariableName=sig_result_002_005  SaveFormat=Structure With Time
  ToWs_Result_Bus_Sig6 : ToWorkspace  VariableName=sig_result_002_006  SaveFormat=Structure With Time
  ToWs_Result_Bus_Sig7 : ToWorkspace  VariableName=sig_result_002_007  SaveFormat=Structure With Time
  ToWs_Result_Bus_Sig8 : ToWorkspace  VariableName=sig_result_002_008  SaveFormat=Structure With Time
  ToWs_Result_Bus_Sig9 : ToWorkspace  VariableName=sig_result_002_009  SaveFormat=Structure With Time
  specifyOutputs : Subsystem
  result : Outport
  wires:
  sig_Req_Bus/1 -> BS/1, specifyOutputs/1(sig_Req_Bus)
  BS/1 -> ToWs_Req_Bus_Sig1/1  "<testSig_PT_trqCrSCurr>"
  BS/2 -> ToWs_Req_Bus_Sig2/1  "<testSig_SpdGov_trqFlt>"
  BS/3 -> ToWs_Req_Bus_Sig3/1  "<testSig_SpdGov_st>"
  BS/4 -> ToWs_Req_Bus_Sig4/1  "<testSig_EngDem_trqInrLim>"
  BS/5 -> ToWs_Req_Bus_Sig5/1  "<testSig_EngDem_trqInrLimLead>"
  BS/6 -> ToWs_Req_Bus_Sig6/1  "<testSig_SpdGov_trqLead>"
  BS/7 -> ToWs_Req_Bus_Sig7/1  "<testSig_PT_trqCrSLead>"
  BS/8 -> ToWs_Req_Bus_Sig8/1  "<testSig_PT_trqCrSDes>"
  BS/9 -> ToWs_Req_Bus_Sig9/1  "<testSig_RngMod_trqCrSMin>"
  BS/10 -> ToWs_Req_Bus_Sig10/1  "<testSig_EngDem_trqInrLimSlow>"
  BS/11 -> ToWs_Req_Bus_Sig11/1  "<testSig_SpdGov_trqSet>"
  BS/12 -> ToWs_Req_Bus_Sig12/1  "<testSig_CoPT_trqDesCompEng>"
  BS/13 -> ToWs_Req_Bus_Sig13/1  "<testSig_CoVeh_trqDesCompNoFl>"
  BS/14 -> ToWs_Req_Bus_Sig14/1  "<testSig_PT_trqCrSPTPrt>"
  BS/15 -> ToWs_Req_Bus_Sig15/1  "<testSig_RngMod_trqMin>"
  BS/16 -> ToWs_Req_Bus_Sig16/1  "<testSig_VMD_stBrkDes>"
  BS/17 -> ToWs_Req_Bus_Sig17/1  "<testSig_CoVMD_trqLLim>"
  BS/18 -> ToWs_Req_Bus_Sig18/1  "<testSig_AccPed_rTrq>"
  BS/19 -> ToWs_Req_Bus_Sig19/1  "<testSig_CoVeh_trqDesCompVeh>"
  BS/20 -> ToWs_Req_Bus_Sig20/1  "<testSig_PT_trqLos>"
  BS/21 -> ToWs_Req_Bus_Sig21/1  "<testSig_CoVeh_trqAcs>"
  BS/22 -> ToWs_Req_Bus_Sig22/1  "<testSig_CoETS_trqTSEAEngMax>"
  BS/23 -> ToWs_Req_Bus_Sig23/1  "<testSig_CoETS_trqTSEAEngMin>"
  BS/24 -> ToWs_Req_Bus_Sig24/1  "<testSig_PT_trqCrSDCS>"
  BS/25 -> ToWs_Req_Bus_Sig25/1  "<testSig_CoETS_trqInrCurr>"
  BS/26 -> ToWs_Req_Bus_Sig26/1  "<testSig_CoETS_trqInrCurrFast>"
  BS/27 -> ToWs_Req_Bus_Sig27/1  "<testSig_CoETS_trqInrLead>"
  BS/28 -> ToWs_Req_Bus_Sig28/1  "<testSig_CoETS_trqInrLeadFast>"
  BS/29 -> ToWs_Req_Bus_Sig29/1  "<testSig_CoETS_stInrDesBrk>"
  BS/30 -> ToWs_Req_Bus_Sig30/1  "<testSig_CoETS_trqSpdGovLim>"
  BS/31 -> ToWs_Req_Bus_Sig31/1  "<testSig_CoETS_trqLlim>"
  BS/32 -> ToWs_Req_Bus_Sig32/1  "<testSig_CoETS_trqInrLtd>"
  BS/33 -> ToWs_Req_Bus_Sig33/1  "<testSig_CoETS_trqUnFltLtd>"
  BS/34 -> ToWs_Req_Bus_Sig34/1  "<testSig_CoETS_trqInrSet_mp>"
  BS/35 -> ToWs_Req_Bus_Sig35/1  "<testSig_CoETS_trqInrSetSlow>"
  BS/36 -> ToWs_Req_Bus_Sig36/1  "<testSig_CoETS_trqUnFltLtdSet>"
  BS/37 -> ToWs_Req_Bus_Sig37/1  "<testSig_CoETS_trqInrLtdPre_mp>"
  BS/38 -> ToWs_Req_Bus_Sig38/1  "<testSig_CoETS_trqUnFltSet>"
  BS/39 -> ToWs_Req_Bus_Sig39/1  "<testSig_CoETS_trqInrLimSet>"
  BS/40 -> ToWs_Req_Bus_Sig40/1  "<testSig_CoETS_trqInrDesNTC>"
  sig_Result_Bus/1 -> BS_Result/1, specifyOutputs/2(sig_Result_Bus)
  BS_Result/1 -> ToWs_Result_Bus_Sig1/1  "<CoETS_trqInrCurr>"
  BS_Result/2 -> ToWs_Result_Bus_Sig2/1  "<CoETS_trqInrCurrFast>"
  BS_Result/3 -> ToWs_Result_Bus_Sig3/1  "<CoETS_trqInrLead>"
  BS_Result/4 -> ToWs_Result_Bus_Sig4/1  "<CoETS_trqInrLeadFast>"
  BS_Result/5 -> ToWs_Result_Bus_Sig5/1  "<CoETS_stInrDesBrk>"
  BS_Result/6 -> ToWs_Result_Bus_Sig6/1  "<CoETS_trqSpdGovLim>"
  BS_Result/7 -> ToWs_Result_Bus_Sig7/1  "<CoETS_trqLlim>"
  BS_Result/8 -> ToWs_Result_Bus_Sig8/1  "<CoETS_trqInrLtd>"
  BS_Result/9 -> ToWs_Result_Bus_Sig9/1  "<CoETS_trqUnFltLtd>"
  BS_Result/10 -> ToWs_Result_Bus_Sig10/1  "<CoETS_trqInrSet_mp>"
  BS_Result/11 -> ToWs_Result_Bus_Sig11/1  "<CoETS_trqInrSetSlow>"
  BS_Result/12 -> ToWs_Result_Bus_Sig12/1  "<CoETS_trqUnFltLtdSet>"
  BS_Result/13 -> ToWs_Result_Bus_Sig13/1  "<CoETS_trqInrLtdPre_mp>"
  BS_Result/14 -> ToWs_Result_Bus_Sig14/1  "<CoETS_trqUnFltSet>"
  BS_Result/15 -> ToWs_Result_Bus_Sig15/1  "<CoETS_trqInrLimSet>"
  BS_Result/16 -> ToWs_Result_Bus_Sig16/1  "<CoETS_trqInrDesNTC>"
  specifyOutputs/1(result) -> result/1

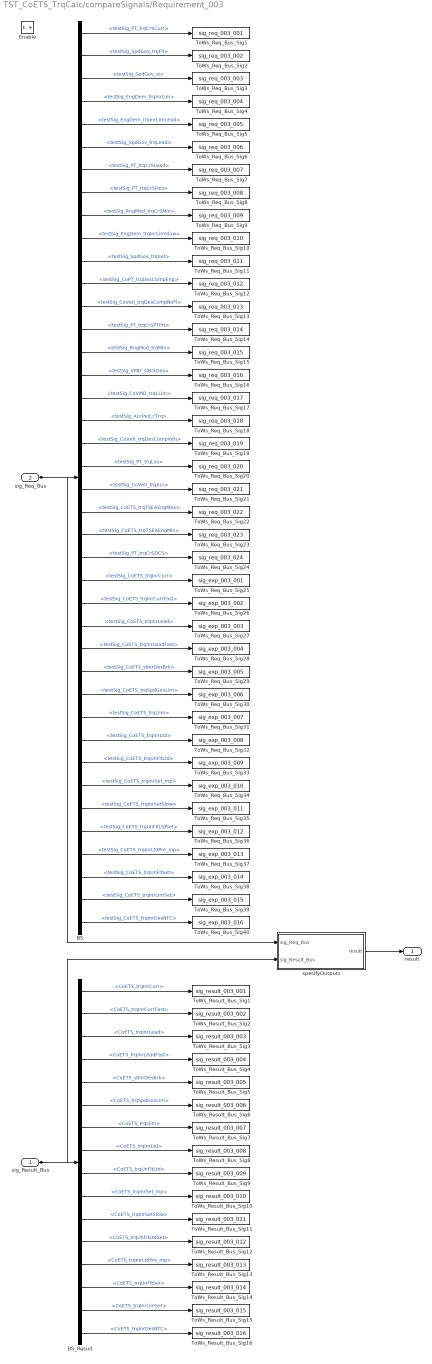
== system TST_CoETS_TrqCalc/compareSignals/Requirement_003 ==
  sig_Result_Bus : Inport
  sig_Req_Bus : Inport  Port=2
  Enable : EnablePort
  BS : BusSelector  OutputSignals=testSig_PT_trqCrSCurr,testSig_SpdGov_trqFlt,testSig_SpdGov_st,testSig_EngDem_trqInrLim,testSig_EngDem_trqInrLimLead,testSig_SpdGov_trqLead,testSig_PT_trqCrSLead,testSig_PT_trqCrSDes,testSig_RngMod_trqCrSMin,testSig_EngDem_trqInrLimSlow,testSig_SpdGov_trqSet,testSig_CoPT_trqDesCompEng,testSig_CoVeh_trqDesCompNoFl,testSig_PT_trqCrSPTPrt,testSig_RngMod_trqMin,testSig_VMD_stBrkDes,testSig_CoVMD_trqLLim,testSig_AccPed_rTrq,testSig_CoVeh_trqDesCompVeh,testSig_PT_trqLos,testSig_CoVeh_trqAcs,testSig_CoETS_trqTSEAEngMax,testSig_CoETS_trqTSEAEngMin,testSig_PT_trqCrSDCS,testSig_CoETS_trqInrCurr,testSig_CoETS_trqInrCurrFast,testSig_CoETS_trqInrLead,testSig_CoETS_trqInrLeadFast,testSig_CoETS_stInrDesBrk,testSig_CoETS_trqSpdGovLim,testSig_CoETS_trqLlim,testSig_CoETS_trqInrLtd,testSig_CoETS_trqUnFltLtd,testSig_CoETS_trqInrSet_mp,testSig_CoETS_trqInrSetSlow,testSig_CoETS_trqUnFltLtdSet,testSig_CoETS_trqInrLtdPre_mp,testSig_CoETS_trqUnFltSet,testSig_CoETS_trqInrLimSet,testSig_CoETS_trqInrDesNTC
  BS_Result : BusSelector  OutputSignals=CoETS_trqInrCurr,CoETS_trqInrCurrFast,CoETS_trqInrLead,CoETS_trqInrLeadFast,CoETS_stInrDesBrk,CoETS_trqSpdGovLim,CoETS_trqLlim,CoETS_trqInrLtd,CoETS_trqUnFltLtd,CoETS_trqInrSet_mp,CoETS_trqInrSetSlow,CoETS_trqUnFltLtdSet,CoETS_trqInrLtdPre_mp,CoETS_trqUnFltSet,CoETS_trqInrLimSet,CoETS_trqInrDesNTC
  ToWs_Req_Bus_Sig1 : ToWorkspace  VariableName=sig_req_003_001  SaveFormat=Structure With Time
  ToWs_Req_Bus_Sig10 : ToWorkspace  VariableName=sig_req_003_010  SaveFormat=Structure With Time
  ToWs_Req_Bus_Sig11 : ToWorkspace  VariableName=sig_req_003_011  SaveFormat=Structure With Time
  ToWs_Req_Bus_Sig12 : ToWorkspace  VariableName=sig_req_003_012  SaveFormat=Structure With Time
  ToWs_Req_Bus_Sig13 : ToWorkspace  VariableName=sig_req_003_013  SaveFormat=Structure With Time
  ToWs_Req_Bus_Sig14 : ToWorkspace  VariableName=sig_req_003_014  SaveFormat=Structure With Time
  ToWs_Req_Bus_Sig15 : ToWorkspace  VariableName=sig_req_003_015  SaveFormat=Structure With Time
  ToWs_Req_Bus_Sig16 : ToWorkspace  VariableName=sig_req_003_016  SaveFormat=Structure With Time
  ToWs_Req_Bus_Sig17 : ToWorkspace  VariableName=sig_req_003_017  SaveFormat=Structure With Time
  ToWs_Req_Bus_Sig18 : ToWorkspace  VariableName=sig_req_003_018  SaveFormat=Structure With Time
  ToWs_Req_Bus_Sig19 : ToWorkspace  VariableName=sig_req_003_019  SaveFormat=Structure With Time
  ToWs_Req_Bus_Sig2 : ToWorkspace  VariableName=sig_req_003_002  SaveFormat=Structure With Time
  ToWs_Req_Bus_Sig20 : ToWorkspace  VariableName=sig_req_003_020  SaveFormat=Structure With Time
  ToWs_Req_Bus_Sig21 : ToWorkspace  VariableName=sig_req_003_021  SaveFormat=Structure With Time
  ToWs_Req_Bus_Sig22 : ToWorkspace  VariableName=sig_req_003_022  SaveFormat=Structure With Time
  ToWs_Req_Bus_Sig23 : ToWorkspace  VariableName=sig_req_003_023  SaveFormat=Structure With Time
  ToWs_Req_Bus_Sig24 : ToWorkspace  VariableName=sig_req_003_024  SaveFormat=Structure With Time
  ToWs_Req_Bus_Sig25 : ToWorkspace  VariableName=sig_exp_003_001  SaveFormat=Structure With Time
  ToWs_Req_Bus_Sig26 : ToWorkspace  VariableName=sig_exp_003_002  SaveFormat=Structure With Time
  ToWs_Req_Bus_Sig27 : ToWorkspace  VariableName=sig_exp_003_003  SaveFormat=Structure With Time
  ToWs_Req_Bus_Sig28 : ToWorkspace  VariableName=sig_exp_003_004  SaveFormat=Structure With Time
  ToWs_Req_Bus_Sig29 : ToWorkspace  VariableName=sig_exp_003_005  SaveFormat=Structure With Time
  ToWs_Req_Bus_Sig3 : ToWorkspace  VariableName=sig_req_003_003  SaveFormat=Structure With Time
  ToWs_Req_Bus_Sig30 : ToWorkspace  VariableName=sig_exp_003_006  SaveFormat=Structure With Time
  ToWs_Req_Bus_Sig31 : ToWorkspace  VariableName=sig_exp_003_007  SaveFormat=Structure With Time
  ToWs_Req_Bus_Sig32 : ToWorkspace  VariableName=sig_exp_003_008  SaveFormat=Structure With Time
  ToWs_Req_Bus_Sig33 : ToWorkspace  VariableName=sig_exp_003_009  SaveFormat=Structure With Time
  ToWs_Req_Bus_Sig34 : ToWorkspace  VariableName=sig_exp_003_010  SaveFormat=Structure With Time
  ToWs_Req_Bus_Sig35 : ToWorkspace  VariableName=sig_exp_003_011  SaveFormat=Structure With Time
  ToWs_Req_Bus_Sig36 : ToWorkspace  VariableName=sig_exp_003_012  SaveFormat=Structure With Time
  ToWs_Req_Bus_Sig37 : ToWorkspace  VariableName=sig_exp_003_013  SaveFormat=Structure With Time
  ToWs_Req_Bus_Sig38 : ToWorkspace  VariableName=sig_exp_003_014  SaveFormat=Structure With Time
  ToWs_Req_Bus_Sig39 : ToWorkspace  VariableName=sig_exp_003_015  SaveFormat=Structure With Time
  ToWs_Req_Bus_Sig4 : ToWorkspace  VariableName=sig_req_003_004  SaveFormat=Structure With Time
  ToWs_Req_Bus_Sig40 : ToWorkspace  VariableName=sig_exp_003_016  SaveFormat=Structure With Time
  ToWs_Req_Bus_Sig5 : ToWorkspace  VariableName=sig_req_003_005  SaveFormat=Structure With Time
  ToWs_Req_Bus_Sig6 : ToWorkspace  VariableName=sig_req_003_006  SaveFormat=Structure With Time
  ToWs_Req_Bus_Sig7 : ToWorkspace  VariableName=sig_req_003_007  SaveFormat=Structure With Time
  ToWs_Req_Bus_Sig8 : ToWorkspace  VariableName=sig_req_003_008  SaveFormat=Structure With Time
  ToWs_Req_Bus_Sig9 : ToWorkspace  VariableName=sig_req_003_009  SaveFormat=Structure With Time
  ToWs_Result_Bus_Sig1 : ToWorkspace  VariableName=sig_result_003_001  SaveFormat=Structure With Time
  ToWs_Result_Bus_Sig10 : ToWorkspace  VariableName=sig_result_003_010  SaveFormat=Structure With Time
  ToWs_Result_Bus_Sig11 : ToWorkspace  VariableName=sig_result_003_011  SaveFormat=Structure With Time
  ToWs_Result_Bus_Sig12 : ToWorkspace  VariableName=sig_result_003_012  SaveFormat=Structure With Time
  ToWs_Result_Bus_Sig13 : ToWorkspace  VariableName=sig_result_003_013  SaveFormat=Structure With Time
  ToWs_Result_Bus_Sig14 : ToWorkspace  VariableName=sig_result_003_014  SaveFormat=Structure With Time
  ToWs_Result_Bus_Sig15 : ToWorkspace  VariableName=sig_result_003_015  SaveFormat=Structure With Time
  ToWs_Result_Bus_Sig16 : ToWorkspace  VariableName=sig_result_003_016  SaveFormat=Structure With Time
  ToWs_Result_Bus_Sig2 : ToWorkspace  VariableName=sig_result_003_002  SaveFormat=Structure With Time
  ToWs_Result_Bus_Sig3 : ToWorkspace  VariableName=sig_result_003_003  SaveFormat=Structure With Time
  ToWs_Result_Bus_Sig4 : ToWorkspace  VariableName=sig_result_003_004  SaveFormat=Structure With Time
  ToWs_Result_Bus_Sig5 : ToWorkspace  VariableName=sig_result_003_005  SaveFormat=Structure With Time
  ToWs_Result_Bus_Sig6 : ToWorkspace  VariableName=sig_result_003_006  SaveFormat=Structure With Time
  ToWs_Result_Bus_Sig7 : ToWorkspace  VariableName=sig_result_003_007  SaveFormat=Structure With Time
  ToWs_Result_Bus_Sig8 : ToWorkspace  VariableName=sig_result_003_008  SaveFormat=Structure With Time
  ToWs_Result_Bus_Sig9 : ToWorkspace  VariableName=sig_result_003_009  SaveFormat=Structure With Time
  specifyOutputs : Subsystem
  result : Outport
  wires:
  sig_Req_Bus/1 -> BS/1, specifyOutputs/1(sig_Req_Bus)
  BS/1 -> ToWs_Req_Bus_Sig1/1  "<testSig_PT_trqCrSCurr>"
  BS/2 -> ToWs_Req_Bus_Sig2/1  "<testSig_SpdGov_trqFlt>"
  BS/3 -> ToWs_Req_Bus_Sig3/1  "<testSig_SpdGov_st>"
  BS/4 -> ToWs_Req_Bus_Sig4/1  "<testSig_EngDem_trqInrLim>"
  BS/5 -> ToWs_Req_Bus_Sig5/1  "<testSig_EngDem_trqInrLimLead>"
  BS/6 -> ToWs_Req_Bus_Sig6/1  "<testSig_SpdGov_trqLead>"
  BS/7 -> ToWs_Req_Bus_Sig7/1  "<testSig_PT_trqCrSLead>"
  BS/8 -> ToWs_Req_Bus_Sig8/1  "<testSig_PT_trqCrSDes>"
  BS/9 -> ToWs_Req_Bus_Sig9/1  "<testSig_RngMod_trqCrSMin>"
  BS/10 -> ToWs_Req_Bus_Sig10/1  "<testSig_EngDem_trqInrLimSlow>"
  BS/11 -> ToWs_Req_Bus_Sig11/1  "<testSig_SpdGov_trqSet>"
  BS/12 -> ToWs_Req_Bus_Sig12/1  "<testSig_CoPT_trqDesCompEng>"
  BS/13 -> ToWs_Req_Bus_Sig13/1  "<testSig_CoVeh_trqDesCompNoFl>"
  BS/14 -> ToWs_Req_Bus_Sig14/1  "<testSig_PT_trqCrSPTPrt>"
  BS/15 -> ToWs_Req_Bus_Sig15/1  "<testSig_RngMod_trqMin>"
  BS/16 -> ToWs_Req_Bus_Sig16/1  "<testSig_VMD_stBrkDes>"
  BS/17 -> ToWs_Req_Bus_Sig17/1  "<testSig_CoVMD_trqLLim>"
  BS/18 -> ToWs_Req_Bus_Sig18/1  "<testSig_AccPed_rTrq>"
  BS/19 -> ToWs_Req_Bus_Sig19/1  "<testSig_CoVeh_trqDesCompVeh>"
  BS/20 -> ToWs_Req_Bus_Sig20/1  "<testSig_PT_trqLos>"
  BS/21 -> ToWs_Req_Bus_Sig21/1  "<testSig_CoVeh_trqAcs>"
  BS/22 -> ToWs_Req_Bus_Sig22/1  "<testSig_CoETS_trqTSEAEngMax>"
  BS/23 -> ToWs_Req_Bus_Sig23/1  "<testSig_CoETS_trqTSEAEngMin>"
  BS/24 -> ToWs_Req_Bus_Sig24/1  "<testSig_PT_trqCrSDCS>"
  BS/25 -> ToWs_Req_Bus_Sig25/1  "<testSig_CoETS_trqInrCurr>"
  BS/26 -> ToWs_Req_Bus_Sig26/1  "<testSig_CoETS_trqInrCurrFast>"
  BS/27 -> ToWs_Req_Bus_Sig27/1  "<testSig_CoETS_trqInrLead>"
  BS/28 -> ToWs_Req_Bus_Sig28/1  "<testSig_CoETS_trqInrLeadFast>"
  BS/29 -> ToWs_Req_Bus_Sig29/1  "<testSig_CoETS_stInrDesBrk>"
  BS/30 -> ToWs_Req_Bus_Sig30/1  "<testSig_CoETS_trqSpdGovLim>"
  BS/31 -> ToWs_Req_Bus_Sig31/1  "<testSig_CoETS_trqLlim>"
  BS/32 -> ToWs_Req_Bus_Sig32/1  "<testSig_CoETS_trqInrLtd>"
  BS/33 -> ToWs_Req_Bus_Sig33/1  "<testSig_CoETS_trqUnFltLtd>"
  BS/34 -> ToWs_Req_Bus_Sig34/1  "<testSig_CoETS_trqInrSet_mp>"
  BS/35 -> ToWs_Req_Bus_Sig35/1  "<testSig_CoETS_trqInrSetSlow>"
  BS/36 -> ToWs_Req_Bus_Sig36/1  "<testSig_CoETS_trqUnFltLtdSet>"
  BS/37 -> ToWs_Req_Bus_Sig37/1  "<testSig_CoETS_trqInrLtdPre_mp>"
  BS/38 -> ToWs_Req_Bus_Sig38/1  "<testSig_CoETS_trqUnFltSet>"
  BS/39 -> ToWs_Req_Bus_Sig39/1  "<testSig_CoETS_trqInrLimSet>"
  BS/40 -> ToWs_Req_Bus_Sig40/1  "<testSig_CoETS_trqInrDesNTC>"
  sig_Result_Bus/1 -> BS_Result/1, specifyOutputs/2(sig_Result_Bus)
  BS_Result/1 -> ToWs_Result_Bus_Sig1/1  "<CoETS_trqInrCurr>"
  BS_Result/2 -> ToWs_Result_Bus_Sig2/1  "<CoETS_trqInrCurrFast>"
  BS_Result/3 -> ToWs_Result_Bus_Sig3/1  "<CoETS_trqInrLead>"
  BS_Result/4 -> ToWs_Result_Bus_Sig4/1  "<CoETS_trqInrLeadFast>"
  BS_Result/5 -> ToWs_Result_Bus_Sig5/1  "<CoETS_stInrDesBrk>"
  BS_Result/6 -> ToWs_Result_Bus_Sig6/1  "<CoETS_trqSpdGovLim>"
  BS_Result/7 -> ToWs_Result_Bus_Sig7/1  "<CoETS_trqLlim>"
  BS_Result/8 -> ToWs_Result_Bus_Sig8/1  "<CoETS_trqInrLtd>"
  BS_Result/9 -> ToWs_Result_Bus_Sig9/1  "<CoETS_trqUnFltLtd>"
  BS_Result/10 -> ToWs_Result_Bus_Sig10/1  "<CoETS_trqInrSet_mp>"
  BS_Result/11 -> ToWs_Result_Bus_Sig11/1  "<CoETS_trqInrSetSlow>"
  BS_Result/12 -> ToWs_Result_Bus_Sig12/1  "<CoETS_trqUnFltLtdSet>"
  BS_Result/13 -> ToWs_Result_Bus_Sig13/1  "<CoETS_trqInrLtdPre_mp>"
  BS_Result/14 -> ToWs_Result_Bus_Sig14/1  "<CoETS_trqUnFltSet>"
  BS_Result/15 -> ToWs_Result_Bus_Sig15/1  "<CoETS_trqInrLimSet>"
  BS_Result/16 -> ToWs_Result_Bus_Sig16/1  "<CoETS_trqInrDesNTC>"
  specifyOutputs/1(result) -> result/1
